simulink model "esercizio_simulink"  (R2023b)
settings: Solver=VariableStepAuto  StartTime=0.0  StopTime=t_sim  RelTol=1e-3
undefined symbols (not defined in the file): x_0_1, x_0_2
settings Model: Creator=alberto  LastModifiedBy=alberto

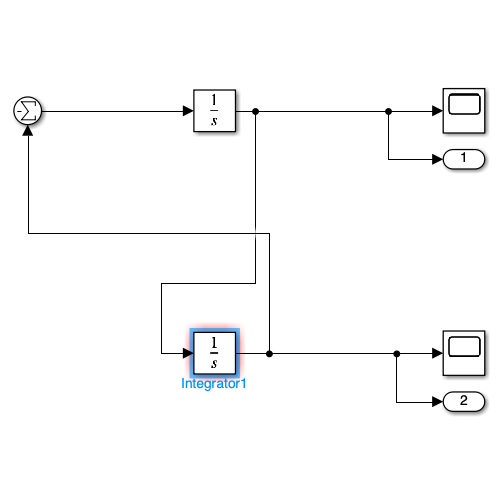
[thumbnail: Simulink's stored preview of the top-level diagram]
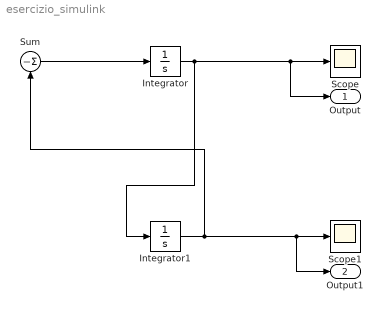
== system esercizio_simulink ==
  Integrator : Integrator  InitialCondition=x_0_1
  Integrator1 : Integrator  InitialCondition=x_0_2
  Scope : Scope
  Scope1 : Scope
  Sum : Sum  Inputs=|-
  Output : Outport
  Output1 : Outport  Port=2
  wires:
  Sum/1 -> Integrator/1
  Integrator1/1 -> Output1/1, Scope1/1, Sum/1
  Integrator/1 -> Output/1, Scope/1, Integrator1/1
